simulink model "model_secours"  (R2022a)
settings: Solver=VariableStepAuto  StartTime=0.0  StopTime=Tf-Ts  RelTol=1e-3
undefined symbols (not defined in the file or in its folder): alpha, biais_sensor, c, gama, M, mdot, R, sigbuilder_block, theta, Ts, Tz_init
libraries: dspsrcs4 x2, dspmathops x1
settings Model: Creator=masdoua1  LastModifiedBy=masdoua1

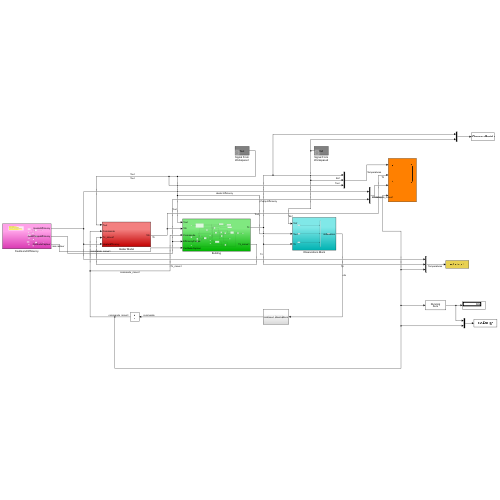
[thumbnail: Simulink's stored preview of the top-level diagram]
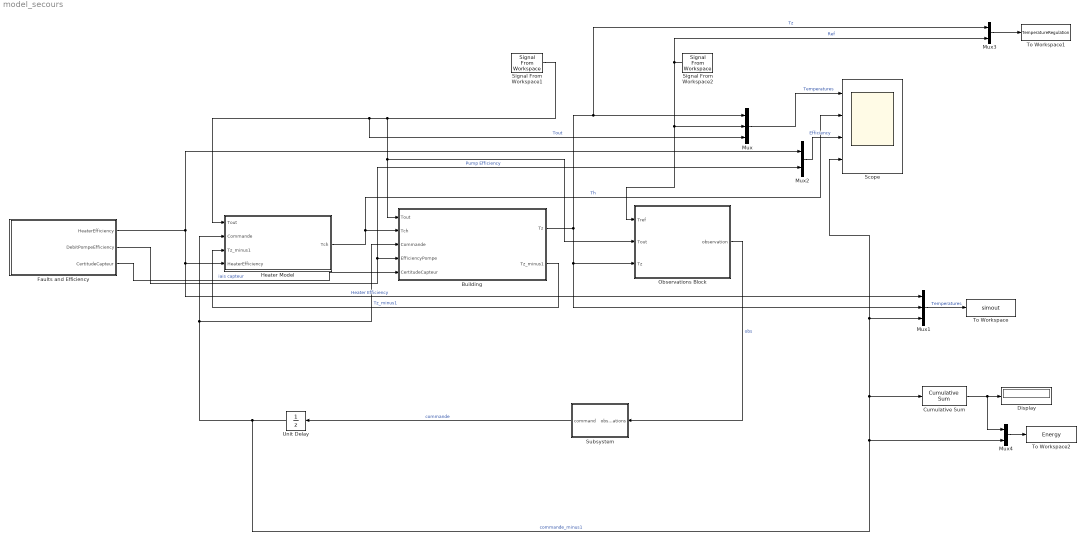
== system model_secours ==
  Building : Subsystem
  Cumulative Sum : dspmathops/Cumulative Sum  dim=Channels (running sum)  InputProcessing=Columns as channels (frame based)  reset_popup=None  roundingMode=Floor  overflowMode=off  outputDataTypeStr=Inherit: Same as accumulator  outputMin=[]  outputMax=[]  outputLastDataTypeStr=Inherit: Same as accumulator
  Display : Display
  Faults and Efficiency : Subsystem
  Heater Model : Subsystem
  Mux : Mux  Inputs=3
  Mux1 : Mux  Inputs=3
  Mux2 : Mux  Inputs=2
  Mux3 : Mux  Inputs=2
  Mux4 : Mux  Inputs=2
  Observations Block : Subsystem
  Scope : Scope  NumInputPorts=4
  Signal From Workspace1 : dspsrcs4/Signal From Workspace  X=Tout  Ts=1  nsamps=1  OutputAfterFinalValue=Setting to zero  ignoreOrWarnInputAndFrameLengths=off  OutputFrames=off
  Signal From Workspace2 : dspsrcs4/Signal From Workspace  X=Ref  Ts=1  nsamps=1  OutputAfterFinalValue=Setting to zero  ignoreOrWarnInputAndFrameLengths=off  OutputFrames=off
  Subsystem : Subsystem
  To Workspace : ToWorkspace  VariableName=simout  SaveFormat=Timeseries  SampleTime=-1
  To Workspace1 : ToWorkspace  VariableName=TemperatureRegulation  SaveFormat=Timeseries  SampleTime=-1
  To Workspace2 : ToWorkspace  VariableName=Energy  SaveFormat=Timeseries  SampleTime=-1
  Unit Delay : UnitDelay  SampleTime=-1  HasFrameUpgradeWarning=on
  wires:
  Unit Delay/1 -> Cumulative Sum/1, Scope/4, Mux1/3, Mux4/2, Heater Model/2(Commande), Building/3(Commande)  "commande_minus1"
  Signal From Workspace2/1 -> Mux3/2, Mux/2, Observations Block/1(Tref)  "Ref"
  Observations Block/1(observation) -> Subsystem/1(observations)  "obs"
  Subsystem/1(command) -> Unit Delay/1  "commande"
  Signal From Workspace1/1 -> Heater Model/1(Tout), Mux/3, Observations Block/2(Tout), Building/1(Tout)  "Tout"
  Building/1(Tz) -> Observations Block/3(Tz), Mux1/2, Mux3/1, Mux/1  "Tz"
  Building/2(Tz_minus1) -> Heater Model/3(Tz_minus1)  "Tz_minus1"
  Heater Model/1(Tch) -> Scope/2, Building/2(Tch)  "Th"
  Mux/1 -> Scope/1  "Temperatures"
  Faults and Efficiency/1(HeaterEfficiency) -> Mux2/1, Heater Model/4(HeaterEfficiency), Mux1/1  "Heater Efficiency"
  Mux1/1 -> To Workspace/1  "Temperatures"
  Faults and Efficiency/2(DebitPompeEfficiency) -> Mux2/2, Building/4(EfficiencyPompe)  "Pump Efficiency"
  Faults and Efficiency/3(CertitudeCapteur) -> Building/5(CertitudeCapteur)  "iais capteur"
  Cumulative Sum/1 -> Mux4/1, Display/1
  Mux2/1 -> Scope/3  "Efficiency"
  Mux3/1 -> To Workspace1/1
  Mux4/1 -> To Workspace2/1

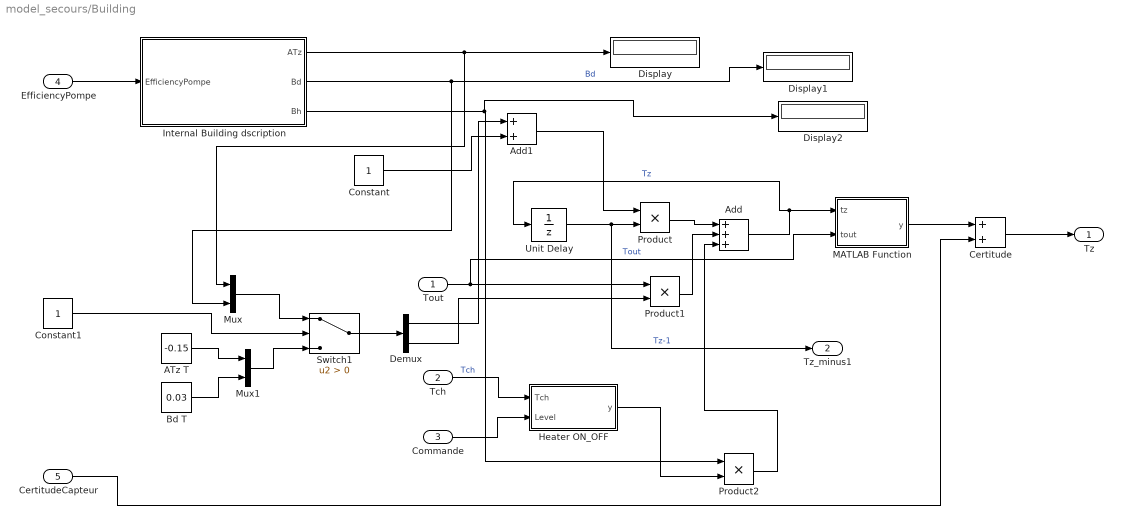
== system model_secours/Building ==
  Tout : Inport
  Tch : Inport  Port=2
  Commande : Inport  Port=3
  EfficiencyPompe : Inport  Port=4
  CertitudeCapteur : Inport  Port=5
  ATz T : Constant  Value=-0.15
  Add : Sum  Inputs=+++
  Add1 : Sum
  Bd T : Constant  Value=0.03
  Certitude : Sum
  Constant : Constant
  Constant1 : Constant
  Demux : Demux  Outputs=2
  Display : Display
  Display1 : Display
  Display2 : Display
  Heater ON_OFF : MATLAB Function  TreatAsAtomicUnit=on
  Internal Building dscription : Subsystem
  MATLAB Function : MATLAB Function  TreatAsAtomicUnit=on
  Mux : Mux  Inputs=2
  Mux1 : Mux  Inputs=2
  Product : Product
  Product1 : Product
  Product2 : Product
  Switch1 : Switch  Criteria=u2 > Threshold  SaturateOnIntegerOverflow=off  InputSameDT=off
  Unit Delay : UnitDelay  InitialCondition=Tz_init  SampleTime=Ts  HasFrameUpgradeWarning=on
  Tz : Outport
  Tz_minus1 : Outport  Port=2
  wires:
  Product/1 -> Add/1
  Unit Delay/1 -> Product/2, Tz_minus1/1  "Tz-1"
  Tout/1 -> Product1/1, MATLAB Function/2(tout)  "Tout"
  Product1/1 -> Add/2
  Add/1 -> Unit Delay/1, MATLAB Function/1(tz)  "Tz"
  Product2/1 -> Add/3
  Commande/1 -> Heater ON_OFF/2(Level)
  Tch/1 -> Heater ON_OFF/1(Tch)  "Tch"
  Heater ON_OFF/1(y) -> Product2/2
  MATLAB Function/1(y) -> Certitude/1
  EfficiencyPompe/1 -> Internal Building dscription/1(EfficiencyPompe)
  Internal Building dscription/1(ATz) -> Mux/1, Display/1
  Constant/1 -> Add1/2
  Add1/1 -> Product/1
  Internal Building dscription/2(Bd) -> Mux/2, Display1/1  "Bd"
  Internal Building dscription/3(Bh) -> Display2/1, Product2/1
  Mux/1 -> Switch1/1
  ATz T/1 -> Mux1/1
  Bd T/1 -> Mux1/2
  Mux1/1 -> Switch1/3
  Switch1/1 -> Demux/1
  Demux/1 -> Add1/1
  Demux/2 -> Product1/2
  Constant1/1 -> Switch1/2
  Certitude/1 -> Tz/1
  CertitudeCapteur/1 -> Certitude/2

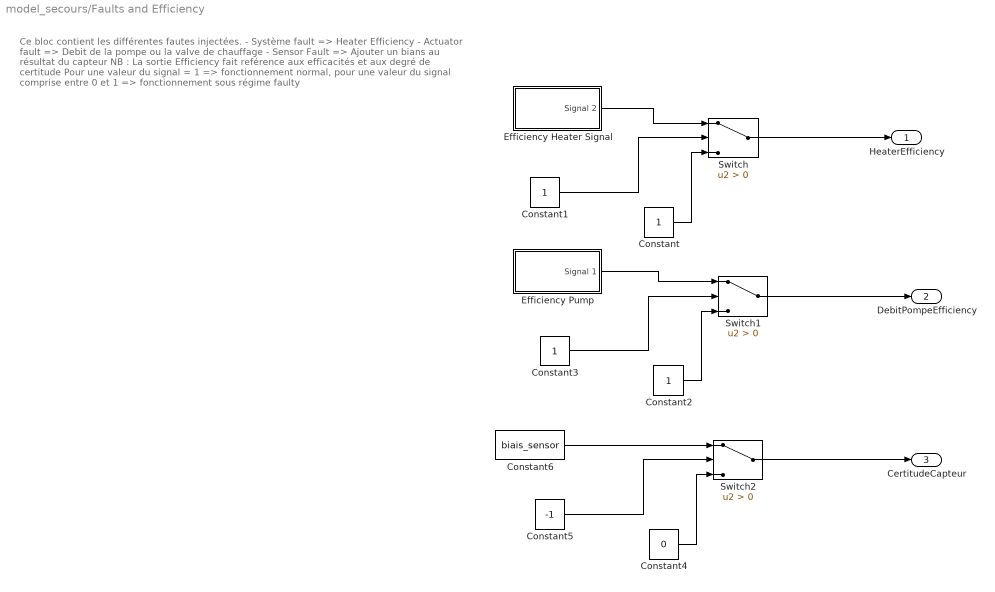
== system model_secours/Faults and Efficiency ==
  note: Ce bloc contient les différentes fautes injectées.
      | - Système fault => Heater Efficiency
      | - Actuator fault => Debit de la pompe ou la valve de chauffage
      | - Sensor Fault => Ajouter un bians au résultat du capteur
      |
      | NB : La sortie Efficiency fait reférence aux efficacités et aux degré de certitude
      | Pour une valeur du signal = 1 => fonctionnement normal, pour une valeur du signal comprise entre 0 et 1 => fonctionnement sous régime faulty
  Constant{,1..3} (4 alike) : Constant
  Constant4 : Constant  Value=0
  Constant5 : Constant  Value=-1
  Constant6 : Constant  Value=biais_sensor
  Efficiency Heater Signal : Subsystem  Tag=STV Subsys  LoadFcn=sigbuilder_block('load');  StartFcn=sigbuilder_block('start');  StopFcn=sigbuilder_block('stop');  ClipboardFcn=sigbuilder_block('clipboard');  mask(Sigbuilder block){tuvar=[0:10]}
      mask help: Simulink:masks:SigbuilderBlock_MD
      mask init:
      | if ~strcmp(get_param(bdroot(gcbh),'SimulationStatus'),'stopped') tuvar = sigbuilder_block('maskInit'); end
      settings: CopyFcn=sigbuilder_block('copy');  DeleteFcn=sigbuilder_block('delete');  ModelCloseFcn=sigbuilder_block('modelClose');  PreSaveFcn=sigbuilder_block('preSave');  PauseFcn=sigbuilder_block('pause');  ContinueFcn=sigbuilder_block('continue');  NameChangeFcn=sigbuilder_block('namechange');  OpenFcn=sigbuilder_block('open',[0 36 1152 555.6 ]);  CloseFcn=sigbuilder_block('close');
      mask Display: plot(0, 0, 100, 100,[2, 2, 32, 32, 2], [68, 8, 8, 68, 68],[32, 2], [38, 38], [32, 19, 2],[53, 60, 44], [32, 17, 17, 2],[16, 16, 31, 31]);txt = getActiveGroup(gcbh);text(2, 100, txt,'verticalAlignment', 'top');
  "Efficiency Pump " : Subsystem  Tag=STV Subsys  LoadFcn=sigbuilder_block('load');  StartFcn=sigbuilder_block('start');  StopFcn=sigbuilder_block('stop');  ClipboardFcn=sigbuilder_block('clipboard');  mask(Sigbuilder block){tuvar=[0:10]}
      mask help: Simulink:masks:SigbuilderBlock_MD
      mask init:
      | if ~strcmp(get_param(bdroot(gcbh),'SimulationStatus'),'stopped') tuvar = sigbuilder_block('maskInit'); end
      settings: CopyFcn=sigbuilder_block('copy');  DeleteFcn=sigbuilder_block('delete');  ModelCloseFcn=sigbuilder_block('modelClose');  PreSaveFcn=sigbuilder_block('preSave');  PauseFcn=sigbuilder_block('pause');  ContinueFcn=sigbuilder_block('continue');  NameChangeFcn=sigbuilder_block('namechange');  OpenFcn=sigbuilder_block('open',[0 36 1152 555.6 ]);  CloseFcn=sigbuilder_block('close');
      mask Display: plot(0, 0, 100, 100,[2, 2, 32, 32, 2], [68, 8, 8, 68, 68],[32, 2], [38, 38], [32, 19, 2],[53, 60, 44], [32, 17, 17, 2],[16, 16, 31, 31]);txt = getActiveGroup(gcbh);text(2, 100, txt,'verticalAlignment', 'top');
  Switch : Switch  Criteria=u2 > Threshold  SaturateOnIntegerOverflow=off  InputSameDT=off
  Switch1 : Switch  Criteria=u2 > Threshold  SaturateOnIntegerOverflow=off  InputSameDT=off
  Switch2 : Switch  Criteria=u2 > Threshold  SaturateOnIntegerOverflow=off  InputSameDT=off
  HeaterEfficiency : Outport
  DebitPompeEfficiency : Outport  Port=2
  CertitudeCapteur : Outport  Port=3
  wires:
  Switch1/1 -> DebitPompeEfficiency/1
  Constant/1 -> Switch/3
  Constant1/1 -> Switch/2
  Switch/1 -> HeaterEfficiency/1
  Constant3/1 -> Switch1/2
  Constant2/1 -> Switch1/3
  Constant5/1 -> Switch2/2
  Constant6/1 -> Switch2/1
  Switch2/1 -> CertitudeCapteur/1
  Constant4/1 -> Switch2/3
  "Efficiency Pump "/1(Signal 1) -> Switch1/1
  Efficiency Heater Signal/1(Signal 2) -> Switch/1

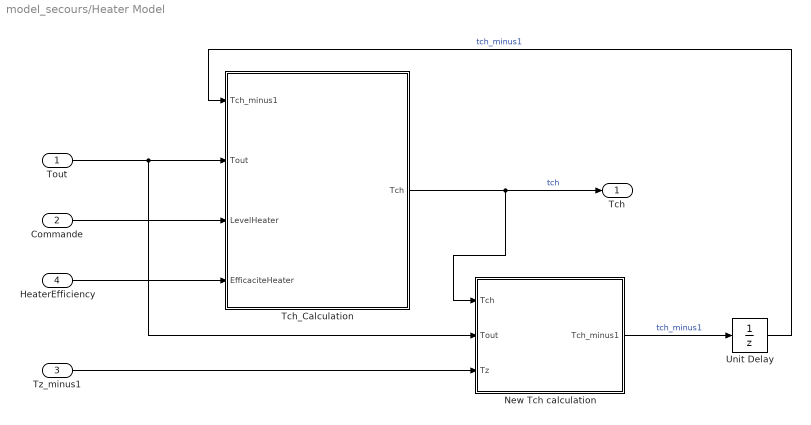
== system model_secours/Heater Model ==
  Tout : Inport
  Commande : Inport  Port=2
  Tz_minus1 : Inport  Port=3
  HeaterEfficiency : Inport  Port=4
  New Tch calculation : Subsystem
  Tch_Calculation : MATLAB Function  TreatAsAtomicUnit=on
  Unit Delay : UnitDelay  SampleTime=-1  HasFrameUpgradeWarning=on
  Tch : Outport
  wires:
  Tout/1 -> Tch_Calculation/2(Tout), New Tch calculation/2(Tout)
  Commande/1 -> Tch_Calculation/3(LevelHeater)
  Tch_Calculation/1(Tch) -> New Tch calculation/1(Tch), Tch/1  "tch"
  Unit Delay/1 -> Tch_Calculation/1(Tch_minus1)  "tch_minus1"
  Tz_minus1/1 -> New Tch calculation/3(Tz)
  New Tch calculation/1(Tch_minus1) -> Unit Delay/1  "tch_minus1"
  HeaterEfficiency/1 -> Tch_Calculation/4(EfficaciteHeater)

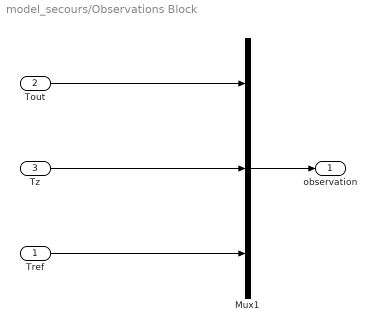
== system model_secours/Observations Block ==
  Tref : Inport
  Tout : Inport  Port=2
  Tz : Inport  Port=3
  Mux1 : Mux  Inputs=3
  observation : Outport
  wires:
  Mux1/1 -> observation/1
  Tz/1 -> Mux1/2
  Tout/1 -> Mux1/1
  Tref/1 -> Mux1/3

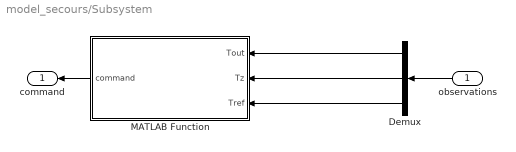
== system model_secours/Subsystem ==
  observations : Inport
  Demux : Demux  Outputs=3
  MATLAB Function : MATLAB Function  TreatAsAtomicUnit=on
  command : Outport
  wires:
  observations/1 -> Demux/1
  Demux/1 -> MATLAB Function/1(Tout)
  Demux/3 -> MATLAB Function/3(Tref)
  MATLAB Function/1(command) -> command/1
  Demux/2 -> MATLAB Function/2(Tz)

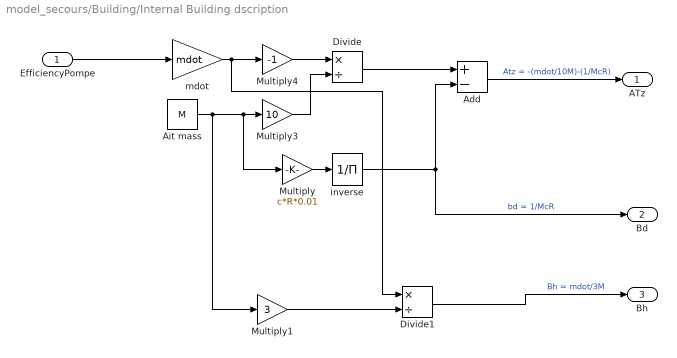
== system model_secours/Building/Internal Building dscription ==
  EfficiencyPompe : Inport
  Add : Sum  Inputs=+-
  Ait mass : Constant  Value=M
  Divide : Product  Inputs=*/
  Divide1 : Product  Inputs=*/
  Multiply : Gain  Gain=c*R*0.01
  Multiply1 : Gain  Gain=3
  Multiply3 : Gain  Gain=10
  Multiply4 : Gain  Gain=-1
  inverse : Product  Inputs=/
  mdot : Gain  Gain=mdot
  ATz : Outport
  Bd : Outport  Port=2
  Bh : Outport  Port=3
  wires:
  Ait mass/1 -> Multiply1/1, Multiply/1, Multiply3/1
  Multiply4/1 -> Divide/1
  Multiply3/1 -> Divide/2
  Divide/1 -> Add/1
  Multiply/1 -> inverse/1
  inverse/1 -> Add/2, Bd/1  "bd = 1/McR"
  Add/1 -> ATz/1  "Atz = -(mdot/10M)-(1/McR)"
  EfficiencyPompe/1 -> mdot/1
  mdot/1 -> Divide1/1, Multiply4/1
  Multiply1/1 -> Divide1/2
  Divide1/1 -> Bh/1  "Bh = mdot/3M"

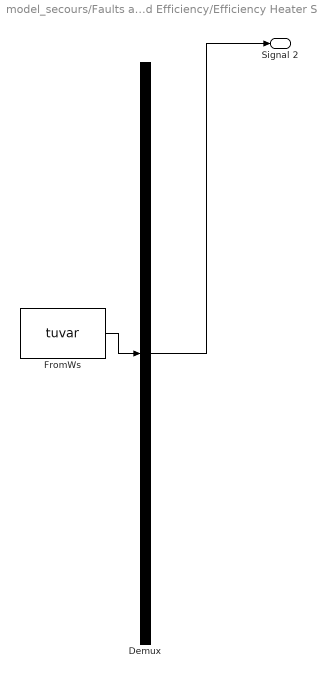
== system model_secours/Faults and Efficiency/Efficiency Heater Signal ==
  Demux : Demux  Tag=STV Demux  Outputs=1
      settings: DisplayOption=none
  FromWs : FromWorkspace  Tag=STV FromWs  VariableName=tuvar
      SigBuilderData=|
      | common.afterFinalStr = 'Extrapolate'
      | common.sampleTime = 0
      | dataSet.timeRange = [0 24]
      | dataSet.name = 'Group 1'
      | sbobj.Groups.Name = 'Group 1'
      | sbobj.Groups.Signals.Name = 'Signal 2'
      | sbobj.Groups.Signals.XData = [0 8 8 16 16 23 24]
      | sbobj.Groups.Signals.YData = [1 1 0.85 0.85 1 1 1]
      | sbobj.Groups.TimeRange = [0 24]
  Signal 2 : Outport  Tag=STV Outport
  wires:
  FromWs/1 -> Demux/1
  Demux/1 -> Signal 2/1

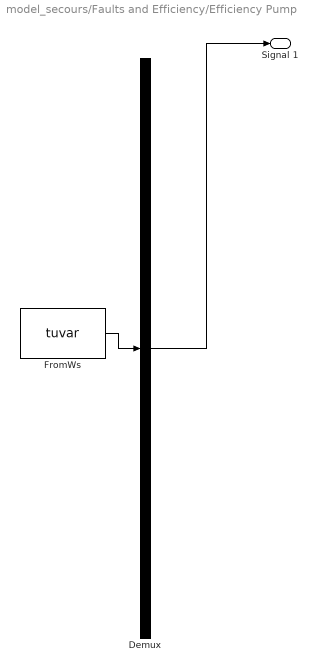
== system model_secours/Faults and Efficiency/Efficiency Pump  ==
  Demux : Demux  Tag=STV Demux  Outputs=1
      settings: DisplayOption=none
  FromWs : FromWorkspace  Tag=STV FromWs  VariableName=tuvar
      SigBuilderData=|
      | common.afterFinalStr = 'Extrapolate'
      | common.sampleTime = 0
      | dataSet.timeRange = [0 24]
      | dataSet.name = 'Group 1'
      | sbobj.Groups.Name = 'Group 1'
      | sbobj.Groups.Signals.Name = 'Signal 1'
      | sbobj.Groups.Signals.XData = [0 10 16 16 24]
      | sbobj.Groups.Signals.YData = [1 1 1 0.85 0.85]
      | sbobj.Groups.TimeRange = [0 24]
  Signal 1 : Outport  Tag=STV Outport
  wires:
  FromWs/1 -> Demux/1
  Demux/1 -> Signal 1/1

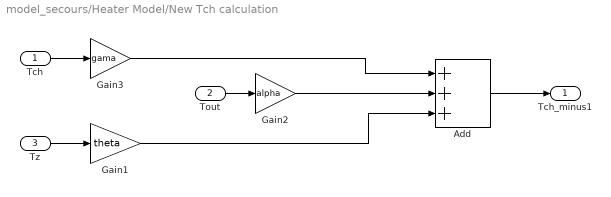
== system model_secours/Heater Model/New Tch calculation ==
  Tch : Inport
  Tout : Inport  Port=2
  Tz : Inport  Port=3
  Add : Sum  Inputs=+++
  Gain1 : Gain  Gain=theta
  Gain2 : Gain  Gain=alpha
  Gain3 : Gain  Gain=gama
  Tch_minus1 : Outport
  wires:
  Add/1 -> Tch_minus1/1
  Gain1/1 -> Add/3
  Tz/1 -> Gain1/1
  Tout/1 -> Gain2/1
  Gain2/1 -> Add/2
  Tch/1 -> Gain3/1
  Gain3/1 -> Add/1

== matlab function model_secours/Heater Model/Tch_Calculation ==
  data: Tch_minus1 input; Tout input; LevelHeater input; Tch output; EfficaciteHeater input
function Tch = fcn(Tch_minus1, Tout, LevelHeater, EfficaciteHeater)
    
    if Tout > Tch_minus1
        Tch_minus1 = Tout+0.2; 
    end
    
    Tch = Tch_minus1 + LevelHeater;
    Tch = Tch*EfficaciteHeater;

== matlab function model_secours/Subsystem/MATLAB Function ==
  data: Tout input; Tz input; command output; Tref input
function command = fcn(Tout, Tz, Tref)

    if Tz < Tref
        command = 7;
    else
    command = 0;
    end
end

== matlab function model_secours/Building/Heater ON_OFF ==
  data: Tch input; Level input; y output
function y = fcn(Tch, Level)
y = Tch;
if Level ==0
        y = 0;
end

== matlab function model_secours/Building/MATLAB Function ==
  data: tz input; tout input; y output
function y = fcn(tz, tout)
y = tz;
    if tz < tout
        y = tout;
    end
